simulink model "STANLEY"  (R2022b)
settings: Solver=ode15s  StartTime=0.0  StopTime=90  FixedStep=0.01  MaxStep=1e-2  MinStep=1e-3  RelTol=5e-3
PreLoadFcn:
  | %centerToFront = 1.4;
  | %centerToRear = 1.4;
values from neighbouring files (symbols this model uses):
  costmap = vehicleCostmap(costmapStruct.Costs,          'FreeThreshold',     costmapStruct.FreeThreshold,          'OccupiedThreshold', costmapStruct.OccupiedThreshold,          'MapLocation',       costmapStruct.MapExtent([1, 3]),          'CellSize',          costmapStruct.CellSize,          'CollisionChecker',  ccConfig)    [VisualizeBicyclePath.m]    (also in createParkingLotCostmap.m = vehicleCostmap(combinedMap,      'CellSize', cellSize,      )
  routePlan = table2struct(routePlan)    [RouteSupervisor.m]
undefined symbols (not defined in the file or in its folder): initialPose
libraries: drivingvehiclecontroller x2, simulink x2, simulink_extras x2, drivinglib x2, autolibshared x1
settings Model: Creator=emanuela  LastModifiedBy=emanuela
settings DataIOCC: SaveFinalState=on  SaveState=on  ReturnWorkspaceOutputs=off

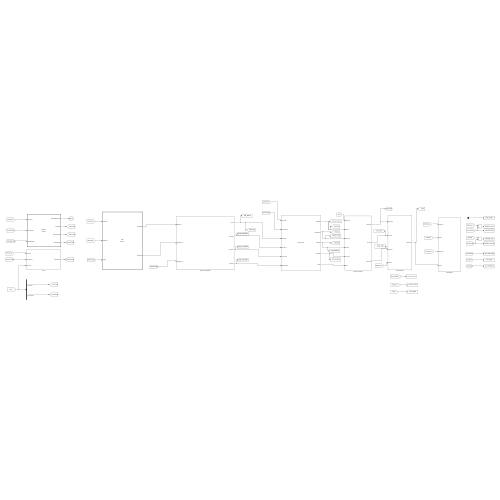
[thumbnail: Simulink's stored preview of the top-level diagram]
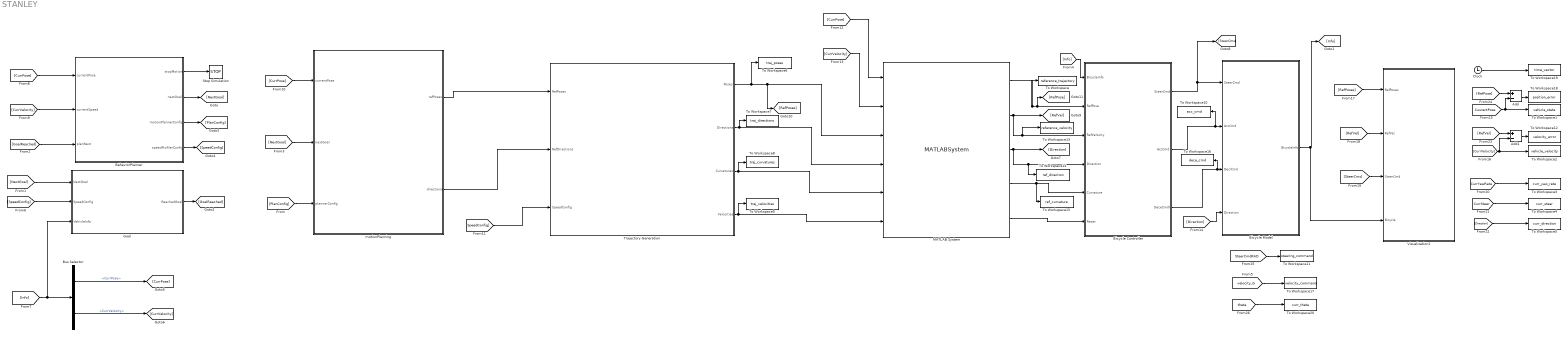
== system STANLEY ==
  Add : Sum  Inputs=+-
  Add1 : Sum  Inputs=+-
  BehaviorPlanner : MATLAB Function  TreatAsAtomicUnit=on  mask{Costmap=costmap, RoutePlan=routePlan, StartSpeed=0}
      mask prompts: Costmap "Vehicle costmap:"; RoutePlan "Route plan:"; StartSpeed "Initial vehicle speed  [m/s]:"
      mask init:
      | validateattributes(Costmap, {'vehicleCostmap'}, {'scalar'});
      | validateattributes(RoutePlan, {'table'}, {'ncols', 3});
      | validateattributes(StartSpeed, {'double'}, {'scalar','nonnegative'})
      | 
      | routePlanStruct   = table2struct(RoutePlan);
      | startPose         = routePlanStruct(1).StartPose;
      | 
      | varagout          = helperSLCreateUtilityStruct(Costmap);
      | vehicleDimsStruct = varagout{1};
      | costmapStruct     = varagout{2};
  Bicycle Controller : Subsystem
  Bicycle Model : Subsystem
  Bus Selector : BusSelector  OutputSignals=CurrPose,CurrVelocity
  Clock : Clock
  Goal : Subsystem
  MATLAB System : MATLABSystem  System=PathTracker  Wheelbase=2.8  HasResetOutput=on  SimulateUsing=Code generation
      mask Type: PathTracker
      mask Display:
      | disp('Path Tracker');
      | port_label('input',1,'CurrPose');
      | port_label('input',2,'CurrVelocity');
      | port_label('input',3,'RefPoses');
      | port_label('input',4,'Directions');
      | port_label('input',5,'Curvatures');
      | port_label('input',6,'RefVelocities');
      | port_label('output',1,'RefPose');
      | port_label('output',2,'RefVelocity');
      | port_label('output',3,'Direction');
      | port_label('output',4,'Curvature');
      | port_label('output',5,'Reset');
  Stop Simulation : Stop
  To Workspace : ToWorkspace  VariableName=reference_trajectory  SaveFormat=Timeseries  SampleTime=-1
  To Workspace1 : ToWorkspace  VariableName=vehicle_state  SaveFormat=Timeseries  SampleTime=-1
  To Workspace10 : ToWorkspace  VariableName=acc_cmd  SaveFormat=Timeseries  SampleTime=-1
  To Workspace11 : ToWorkspace  VariableName=steering_command  SaveFormat=Timeseries  SampleTime=-1
  To Workspace12 : ToWorkspace  VariableName=velocity_error  SaveFormat=Timeseries  SampleTime=-1
  To Workspace13 : ToWorkspace  VariableName=reference_velocity  SaveFormat=Timeseries  SampleTime=-1
  To Workspace14 : ToWorkspace  VariableName=ref_direction  SaveFormat=Timeseries  SampleTime=-1
  To Workspace15 : ToWorkspace  VariableName=ref_curvature  SaveFormat=Timeseries  SampleTime=-1
  To Workspace16 : ToWorkspace  VariableName=dece_cmd  SaveFormat=Timeseries  SampleTime=-1
  To Workspace17 : ToWorkspace  VariableName=velocity_command  SaveFormat=Timeseries  SampleTime=-1
  To Workspace18 : ToWorkspace  VariableName=position_error  SaveFormat=Timeseries  SampleTime=-1
  To Workspace19 : ToWorkspace  VariableName=time_vector  SampleTime=-1
  To Workspace2 : ToWorkspace  VariableName=vehicle_velocity  SaveFormat=Timeseries  SampleTime=-1
  To Workspace20 : ToWorkspace  VariableName=curr_theta  SaveFormat=Timeseries  SampleTime=-1
  To Workspace3 : ToWorkspace  VariableName=curr_yaw_rate  SaveFormat=Timeseries  SampleTime=-1
  To Workspace4 : ToWorkspace  VariableName=curr_steer  SaveFormat=Timeseries  SampleTime=-1
  To Workspace5 : ToWorkspace  VariableName=curr_direction  SaveFormat=Timeseries  SampleTime=-1
  To Workspace6 : ToWorkspace  VariableName=traj_poses  SaveFormat=Timeseries  SampleTime=-1
  To Workspace7 : ToWorkspace  VariableName=traj_directions  SaveFormat=Timeseries  SampleTime=-1
  To Workspace8 : ToWorkspace  VariableName=traj_curvatures  SaveFormat=Timeseries  SampleTime=-1
  To Workspace9 : ToWorkspace  VariableName=traj_velocities  SaveFormat=Timeseries  SampleTime=-1
  Trajectory Generation : Subsystem
  Visualization1 : Subsystem  mask{Costmap=costmap}
      mask prompts: Costmap "Vehicle costmap:"
      mask init:
      | validateattributes(Costmap, {'vehicleCostmap'}, {'scalar'});
      | 
      | varagout          = helperSLCreateUtilityStruct(Costmap);
      | vehicleDimsStruct = varagout{1};
      | costmapStruct     = varagout{2};
      mask DialogControl DescTextVar Prompt: Visualize simulation results.
  motionPlanning : MATLAB Function  TreatAsAtomicUnit=on  mask{Costmap=costmap}
      mask prompts: Costmap "Vehicle costmap:"
      mask init:
      | validateattributes(Costmap, {'vehicleCostmap'}, {'scalar'});
      | 
      | varagout          = helperSLCreateUtilityStruct(Costmap);
      | vehicleDimsStruct = varagout{1};
      | costmapStruct     = varagout{2};
  wires:
  Bicycle Model/1(BicycleInfo) -> Visualization1/4(Bicycle), [Info]
  [Info] -> Bicycle Controller/1(BicycleInfo)
  [NextGoal] -> Goal/1(NextGoal)
  BehaviorPlanner/2(nextGoal) -> [NextGoal]
  BehaviorPlanner/1(stopMotion) -> Stop Simulation/1
  [GoalReached] -> BehaviorPlanner/3(planNext)
  Goal/1(ReachedGoal) -> [GoalReached]
  [NextGoal] -> motionPlanning/2(nextGoal)
  BehaviorPlanner/3(motionPlannerConfig) -> [PlanConfig]
  [PlanConfig] -> motionPlanning/3(plannerConfig)
  BehaviorPlanner/4(speedProfilerConfig) -> [SpeedConfig]
  [SpeedConfig] -> Goal/2(SpeedConfig)
  Bus Selector/1 -> [CurrPose]  "<CurrPose>"
  Bus Selector/2 -> [CurrVelocity]  "<CurrVelocity>"
  [Info] -> Goal/3(VehicleInfo), Bus Selector/1
  [CurrPose] -> BehaviorPlanner/1(currentPose)
  [CurrVelocity] -> BehaviorPlanner/2(currentSpeed)
  [CurrPose] -> motionPlanning/1(currentPose)
  motionPlanning/1(refPoses) -> Trajectory Generation/1(RefPoses)
  motionPlanning/2(directions) -> Trajectory Generation/2(RefDirections)
  [SpeedConfig] -> Trajectory Generation/3(SpeedConfig)
  [CurrPose] -> MATLAB System/1
  [CurrVelocity] -> MATLAB System/2
  Trajectory Generation/2(Directions) -> To Workspace7/1, MATLAB System/4
  Trajectory Generation/3(Curvatures) -> To Workspace8/1, MATLAB System/5
  Trajectory Generation/4(Velocities) -> To Workspace9/1, MATLAB System/6
  MATLAB System/1 -> Bicycle Controller/2(RefPose), [RefPose], To Workspace/1
  MATLAB System/2 -> To Workspace13/1, Bicycle Controller/3(RefVelocity), [RefVel]
  MATLAB System/3 -> [Direction], To Workspace14/1, Bicycle Controller/4(Direction)
  MATLAB System/4 -> To Workspace15/1, Bicycle Controller/5(Curvature)
  Bicycle Controller/1(SteerCmd) -> [SteerCms], Bicycle Model/1(SteerCmd)
  Bicycle Controller/2(AccCmd) -> To Workspace10/1, Bicycle Model/2(AccCmd)
  Bicycle Controller/3(DeceCmdl) -> To Workspace16/1, Bicycle Model/3(DeclCmd)
  [Direction] -> Bicycle Model/4(Direction)
  Trajectory Generation/1(Poses) -> To Workspace6/1, [RefPoses], MATLAB System/3
  MATLAB System/5 -> Bicycle Controller/6(Reset)
  [RefPoses] -> Visualization1/1(RefPoses)
  [RefVel] -> Visualization1/2(RefVel)
  [SteerCms] -> Visualization1/3(SteerCmd)
  [CuurentPose] -> Add/2, To Workspace1/1
  [CurrVelocity] -> Add1/2, To Workspace2/1
  [CurrYawRate] -> To Workspace3/1
  [CurrSteer] -> To Workspace4/1
  [Direction] -> To Workspace5/1
  [RefVel] -> Add1/1
  [RefPose] -> Add/1
  Add1/1 -> To Workspace12/1
  Add/1 -> To Workspace18/1
  Clock/1 -> To Workspace19/1
  [SteerCmdRAD] -> To Workspace11/1
  [velocity_G] -> To Workspace17/1
  [theta] -> To Workspace20/1

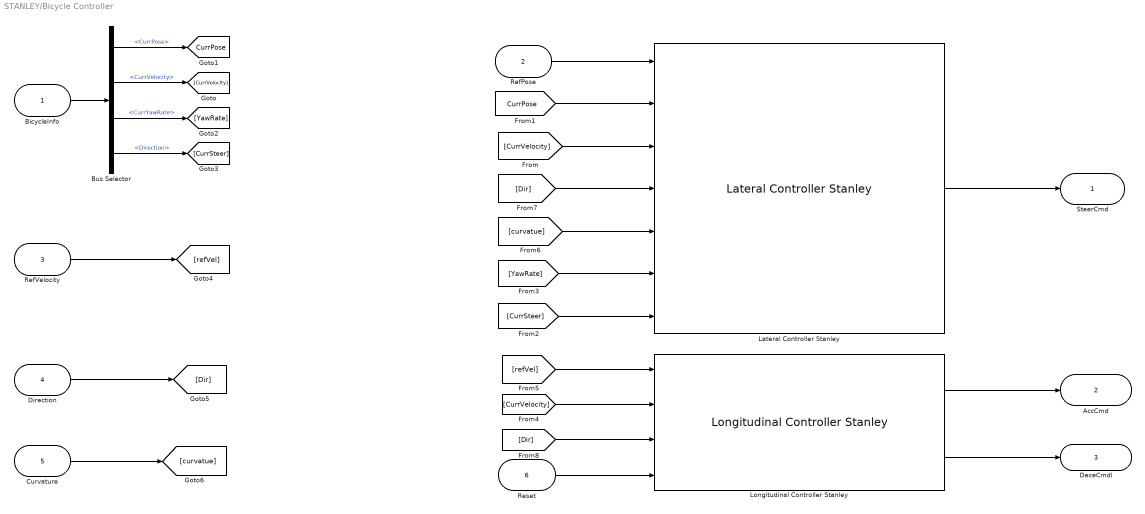
== system STANLEY/Bicycle Controller ==
  BicycleInfo : Inport
  RefPose : Inport  Port=2
  RefVelocity : Inport  Port=3
  Direction : Inport  Port=4
  Curvature : Inport  Port=5
  Reset : Inport  Port=6
  Bus Selector : BusSelector  OutputSignals=CurrPose,CurrVelocity,CurrYawRate,Direction
  Lateral Controller Stanley : drivingvehiclecontroller/Lateral Controller Stanley  ModelType=Dynamic bicycle model  PositionGainF=2  PositionGainR=2.5  YawRateGain=0.25  DelayGain=0.2  VehicleMass=1575  Lf=1.4  Lr=1.4  TireStiffness=19000  Wheelbase=2.8  MaxSteeringAngle=35
  Longitudinal Controller Stanley : drivingvehiclecontroller/Longitudinal Controller Stanley  Kp=2.5  Ki=1  SampleTime=0.01  MaxAcceleration=3  MaxDeceleration=6
  SteerCmd : Outport
  AccCmd : Outport  Port=2
  DeceCmdl : Outport  Port=3
  tag scope: CurrPose=global
  wires:
  BicycleInfo/1 -> Bus Selector/1
  Reset/1 -> Longitudinal Controller Stanley/4
  Lateral Controller Stanley/1 -> SteerCmd/1
  [CurrPose] -> Lateral Controller Stanley/2
  [YawRate] -> Lateral Controller Stanley/6
  [refVel] -> Longitudinal Controller Stanley/1
  [curvatue] -> Lateral Controller Stanley/5
  Longitudinal Controller Stanley/1 -> AccCmd/1
  Longitudinal Controller Stanley/2 -> DeceCmdl/1
  Bus Selector/1 -> [CurrPose]  "<CurrPose>"
  Bus Selector/2 -> [CurrVelocity]  "<CurrVelocity>"
  Bus Selector/3 -> [YawRate]  "<CurrYawRate>"
  Bus Selector/4 -> [CurrSteer]  "<Direction>"
  [CurrSteer] -> Lateral Controller Stanley/7
  [CurrVelocity] -> Lateral Controller Stanley/3
  [CurrVelocity] -> Longitudinal Controller Stanley/2
  RefVelocity/1 -> [refVel]
  Direction/1 -> [Dir]
  [Dir] -> Lateral Controller Stanley/4
  [Dir] -> Longitudinal Controller Stanley/3
  Curvature/1 -> [curvatue]
  RefPose/1 -> Lateral Controller Stanley/1

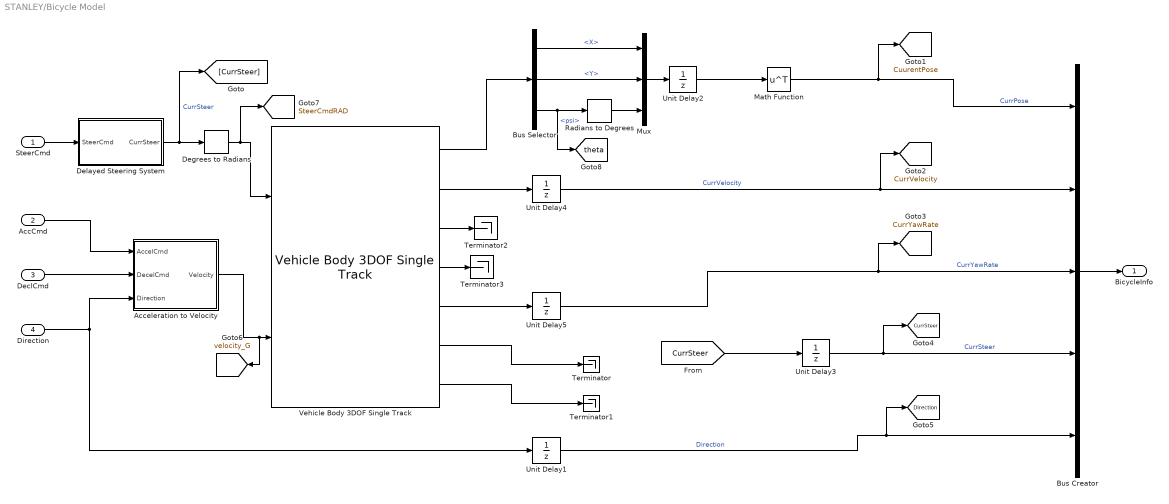
== system STANLEY/Bicycle Model ==
  SteerCmd : Inport
  AccCmd : Inport  Port=2
  DeclCmd : Inport  Port=3
  Direction : Inport  Port=4
  Acceleration to Velocity : Subsystem  TreatAsAtomicUnit=on
  Bus Creator : BusCreator  Inputs=5  OutDataTypeStr=Bus: vehicleInfoBus  NonVirtualBus=on
  Bus Selector : BusSelector  OutputSignals=InertFrm.RearAxl.Disp.X,InertFrm.RearAxl.Disp.Y,InertFrm.Cg.Ang.psi
  Degrees to Radians : simulink_extras/Transformations/Degrees to Radians
  Delayed Steering System : Subsystem
  Math Function : Math  Operator=transpose  SignedPower=on
  Mux : Mux  Inputs=3
  Radians to Degrees : simulink_extras/Transformations/Radians to Degrees
  Terminator{,1..3} (4 alike) : Terminator
  Unit Delay1 : UnitDelay  InitialCondition=1  SampleTime=-1  HasFrameUpgradeWarning=on
  Unit Delay2 : UnitDelay  InitialCondition=initialPose  SampleTime=-1  HasFrameUpgradeWarning=on
  Unit Delay3 : UnitDelay  SampleTime=-1  HasFrameUpgradeWarning=on
  Unit Delay4 : UnitDelay  SampleTime=-1  HasFrameUpgradeWarning=on
  Unit Delay5 : UnitDelay  SampleTime=-1  HasFrameUpgradeWarning=on
  Vehicle Body 3DOF Single Track : autolibshared/Vehicle Body 3DOF Single Track  trackMode=Single (bicycle)  inputMode=External longitudinal velocity  frontSteerMode=on  rearSteerMode=off  windMode=off  muMode=off  extFMode=off  extMMode=off  htchFMode=off  htchMMode=off  extXo=off  extpsio=off  extxdoto=off  extro=off  extYo=off  extTamb=off  extydoto=off  aMode=2  NF=2  NR=2  m=2000  a=1.4  b=1.6  h=0.35  dh=1  hh=0.2  X_o=13.1500  xdot_o=0  CalphaMode=off  sigmaMode=on  d=0  hl=0  w=[1.4,1.4]  Cy_f=12e3  Cy_r=11e3  sigma_f=.1  sigma_r=.1  alpha_f_brk=[-.1 .1]  Cy_f_data=[-9e3 9e3]  alpha_r_brk=[-.1 .1]  Cy_r_data=[-9e3 9e3]  Y_o=93.6500  ydot_o=0  Izz=4000  psi_o=0  r_o=0  Af=2  Cd=.3  Cl=.1  Cpm=.1  beta_w=[0 0.01:0.01:0.3]  Cs=[0 0.01:0.01:0.3]  Cym=[0 1e-6:0.01:0.3]  Pabs=101325  Tair=273  g=9.81  mu=1  xdot_tol=.01  Fznom=5000  Fxtire_sat=7e4  Fytire_sat=7e4  longOff=0  latOff=0  vertOff=0  wrapAng=off
  BicycleInfo : Outport  VectorParamsAs1DForOutWhenUnconnected=off
  tag scope: CurrSteer=global, CurrVelocity=global, CurrYawRate=global, CuurentPose=global, Direction=global, SteerCmdRAD=global, theta=global, velocity_G=global
  wires:
  Vehicle Body 3DOF Single Track/6 -> Terminator/1
  Vehicle Body 3DOF Single Track/7 -> Terminator1/1
  SteerCmd/1 -> Delayed Steering System/1(SteerCmd)
  Delayed Steering System/1(CurrSteer) -> [CurrSteer], Degrees to Radians/1  "CurrSteer"
  Degrees to Radians/1 -> [SteerCmdRAD], Vehicle Body 3DOF Single Track/1
  AccCmd/1 -> Acceleration to Velocity/1(AccelCmd)
  DeclCmd/1 -> Acceleration to Velocity/2(DecelCmd)
  Acceleration to Velocity/1(Velocity) -> [velocity_G], Vehicle Body 3DOF Single Track/2
  Vehicle Body 3DOF Single Track/1 -> Bus Selector/1
  Bus Selector/2 -> Mux/2  "<Y>"
  Unit Delay2/1 -> Math Function/1
  Bus Selector/1 -> Mux/1  "<X>"
  Mux/1 -> Unit Delay2/1
  Math Function/1 -> [CuurentPose], Bus Creator/1  "CurrPose"
  Bus Selector/3 -> [theta], Radians to Degrees/1  "<psi>"
  Radians to Degrees/1 -> Mux/3
  Vehicle Body 3DOF Single Track/3 -> Terminator2/1
  Vehicle Body 3DOF Single Track/2 -> Unit Delay4/1
  Vehicle Body 3DOF Single Track/4 -> Terminator3/1
  Vehicle Body 3DOF Single Track/5 -> Unit Delay5/1
  Direction/1 -> Unit Delay1/1, Acceleration to Velocity/3(Direction)
  Bus Creator/1 -> BicycleInfo/1
  [CurrSteer] -> Unit Delay3/1
  Unit Delay4/1 -> [CurrVelocity], Bus Creator/2  "CurrVelocity"
  Unit Delay5/1 -> [CurrYawRate], Bus Creator/3  "CurrYawRate"
  Unit Delay1/1 -> [Direction], Bus Creator/5  "Direction"
  Unit Delay3/1 -> [CurrSteer], Bus Creator/4  "CurrSteer"

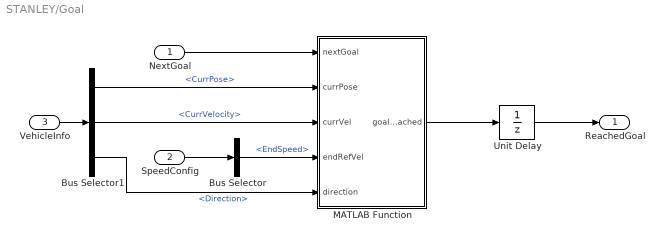
== system STANLEY/Goal ==
  NextGoal : Inport
  SpeedConfig : Inport  Port=2
  VehicleInfo : Inport  Port=3
  Bus Selector : BusSelector  OutputSignals=EndSpeed
  Bus Selector1 : BusSelector  OutputSignals=CurrPose,CurrVelocity,Direction
  MATLAB Function : MATLAB Function  TreatAsAtomicUnit=on
  Unit Delay : UnitDelay  SampleTime=-1  HasFrameUpgradeWarning=on
  ReachedGoal : Outport  VectorParamsAs1DForOutWhenUnconnected=off
  wires:
  Bus Selector/1 -> MATLAB Function/4(endRefVel)  "<EndSpeed>"
  Bus Selector1/1 -> MATLAB Function/2(currPose)  "<CurrPose>"
  VehicleInfo/1 -> Bus Selector1/1
  Unit Delay/1 -> ReachedGoal/1
  Bus Selector1/2 -> MATLAB Function/3(currVel)  "<CurrVelocity>"
  MATLAB Function/1(goalReached) -> Unit Delay/1
  SpeedConfig/1 -> Bus Selector/1
  Bus Selector1/3 -> MATLAB Function/5(direction)  "<Direction>"
  NextGoal/1 -> MATLAB Function/1(nextGoal)

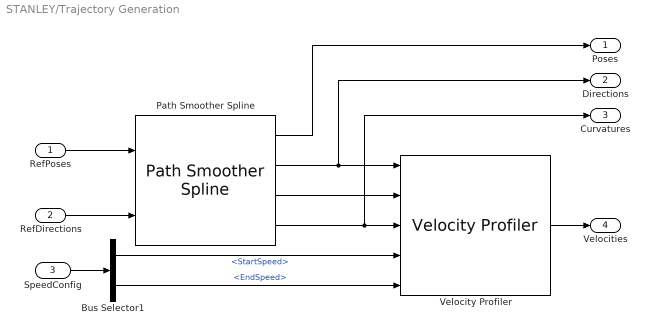
== system STANLEY/Trajectory Generation ==
  RefPoses : Inport
  RefDirections : Inport  Port=2
  SpeedConfig : Inport  Port=3
  Bus Selector1 : BusSelector  OutputSignals=StartSpeed,EndSpeed
  Path Smoother Spline : drivinglib/Path Smoother Spline  NumSmoothPoses=500  MinSeparation=1e-3  SampleTime=-1  ShowOptionalOutports=on  SimulateUsing=Interpreted execution
  Velocity Profiler : drivinglib/Velocity Profiler  MaxLongitudinalAccel=2  MaxLongitudinalDecel=4  MaxSpeed=10  MaxLongitudinalJerk=1  MaxLateralAccel=2  ShowOptionalOutport=off  SampleTime=-1  SimulateUsing=Interpreted execution
  Poses : Outport  VectorParamsAs1DForOutWhenUnconnected=off
  Directions : Outport  Port=2  VectorParamsAs1DForOutWhenUnconnected=off
  Curvatures : Outport  Port=3  VectorParamsAs1DForOutWhenUnconnected=off
  Velocities : Outport  Port=4  VectorParamsAs1DForOutWhenUnconnected=off
  wires:
  Velocity Profiler/1 -> Velocities/1
  Path Smoother Spline/2 -> Directions/1, Velocity Profiler/1
  Path Smoother Spline/4 -> Curvatures/1, Velocity Profiler/3
  Bus Selector1/2 -> Velocity Profiler/5  "<EndSpeed>"
  RefPoses/1 -> Path Smoother Spline/1
  SpeedConfig/1 -> Bus Selector1/1
  Bus Selector1/1 -> Velocity Profiler/4  "<StartSpeed>"
  Path Smoother Spline/3 -> Velocity Profiler/2
  RefDirections/1 -> Path Smoother Spline/2
  Path Smoother Spline/1 -> Poses/1

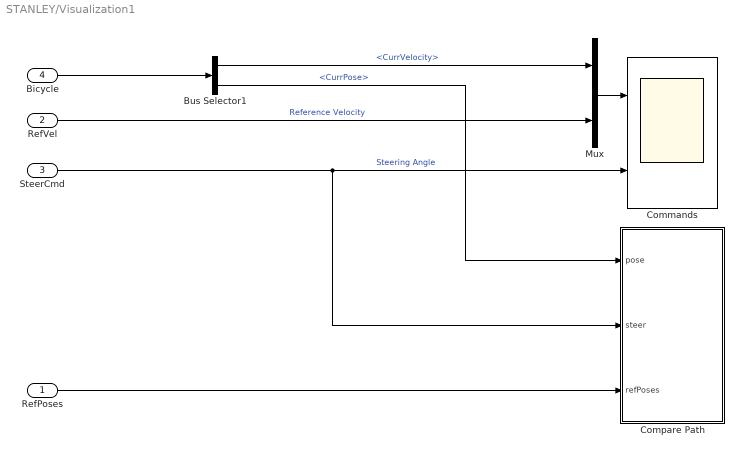
== system STANLEY/Visualization1 ==
  RefPoses : Inport
  RefVel : Inport  Port=2
  SteerCmd : Inport  Port=3
  Bicycle : Inport  Port=4
  Bus Selector1 : BusSelector  OutputSignals=CurrVelocity,CurrPose
  Commands : Scope  NumInputPorts=2
  Compare Path : MATLAB Function  TreatAsAtomicUnit=on
  Mux : Mux  Inputs=2
  wires:
  RefPoses/1 -> Compare Path/3(refPoses)
  Bus Selector1/1 -> Mux/1  "<CurrVelocity>"
  Bus Selector1/2 -> Compare Path/1(pose)  "<CurrPose>"
  RefVel/1 -> Mux/2  "Reference Velocity"
  Mux/1 -> Commands/1
  SteerCmd/1 -> Compare Path/2(steer), Commands/2  "Steering Angle"
  Bicycle/1 -> Bus Selector1/1

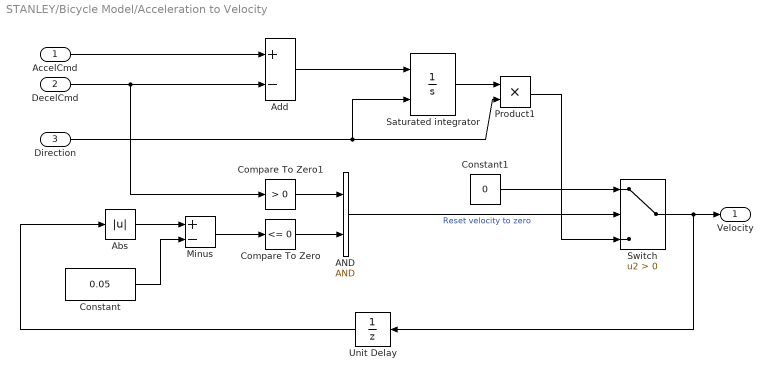
== system STANLEY/Bicycle Model/Acceleration to Velocity ==
  AccelCmd : Inport  PortDimensions=[1 1]
  DecelCmd : Inport  Port=2  PortDimensions=[1 1]
  Direction : Inport  Port=3
  AND : Logic  IconShape=distinctive  AllPortsSameDT=off  OutDataTypeStr=boolean
  Abs : Abs  SaturateOnIntegerOverflow=off
  Add : Sum  Inputs=+-
  Compare To Zero : simulink/Logic and Bit Operations/Compare To Zero  relop=<=  OutDataTypeStr=boolean
  Compare To Zero1 : simulink/Logic and Bit Operations/Compare To Zero  relop=>  OutDataTypeStr=boolean
  Constant : Constant  Value=0.05
  Constant1 : Constant  Value=0
  Minus : Sum  Inputs=+-
  Product1 : Product
  Saturated integrator : Integrator  ExternalReset=either  LimitOutput=on  LowerSaturationLimit=0  AbsoluteTolerance=1e-3  ZeroCross=off
  Switch : Switch  Criteria=u2 > Threshold  SaturateOnIntegerOverflow=off  InputSameDT=off
  Unit Delay : UnitDelay  SampleTime=-1  HasFrameUpgradeWarning=on
  Velocity : Outport  VectorParamsAs1DForOutWhenUnconnected=off
  wires:
  Direction/1 -> Product1/2, Saturated integrator/2
  AccelCmd/1 -> Add/1
  Add/1 -> Saturated integrator/1
  DecelCmd/1 -> Compare To Zero1/1, Add/2
  Unit Delay/1 -> Abs/1
  Abs/1 -> Minus/1
  Constant/1 -> Minus/2
  Minus/1 -> Compare To Zero/1
  Compare To Zero/1 -> AND/2
  Compare To Zero1/1 -> AND/1
  AND/1 -> Switch/2  "Reset velocity to zero"
  Switch/1 -> Unit Delay/1, Velocity/1
  Constant1/1 -> Switch/1
  Saturated integrator/1 -> Product1/1
  Product1/1 -> Switch/3

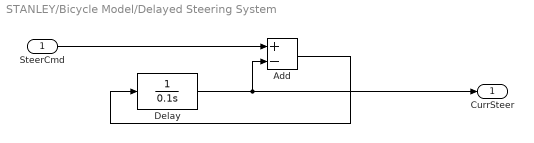
== system STANLEY/Bicycle Model/Delayed Steering System ==
  SteerCmd : Inport
  Add : Sum  Inputs=+-
  Delay : TransferFcn  Denominator=[0.1 0]
  CurrSteer : Outport  VectorParamsAs1DForOutWhenUnconnected=off
  wires:
  Add/1 -> Delay/1
  SteerCmd/1 -> Add/1
  Delay/1 -> CurrSteer/1, Add/2

== matlab function STANLEY/Visualization1/Compare Path ==
  settings: updateMethod=DISCRETE  sampleTime=0.1
  data: pose input size=[1 3]; steer input; refPoses input; costmapStruct parameter; vehicleDimsStruct parameter
function visualizePath(pose, steer, refPoses, costmapStruct, vehicleDimsStruct)

%visualizePath Display simulation results.

coder.extrinsic('VisualizeBicyclePath');

VisualizeBicyclePath(pose, steer, refPoses, costmapStruct, vehicleDimsStruct);
end

== matlab function STANLEY/motionPlanning ==
  settings: updateMethod=DISCRETE  sampleTime=0.1
  data: refPoses output size=[100 3]; currentPose input size=[1 3]; nextGoal input size=[1 3]; plannerConfig input Bus: plannerConfigBus; costmapStruct parameter; vehicleDimsStruct parameter; directions output size=[100 1]
function [refPoses, directions] = motionPlanning(currentPose, nextGoal, ...
    plannerConfig, costmapStruct, vehicleDimsStruct)

%motionPlanning plan a feasible path using pathPlannerRRT.

%#codegen

persistent nextGoalPose posesInternal directionsInternal

% Initialize persistent variables
if isempty(nextGoalPose)
    nextGoalPose = [0 0 0];
end

if isempty(posesInternal)
    posesInternal = [0 0 0];
end

if isempty(directionsInternal)
    directionsInternal = 1;
end

% Create vehicleDimensions object
vehicleDims = vehicleDimensions( ...
    vehicleDimsStruct.Length, ...
    vehicleDimsStruct.Width, ...
    vehicleDimsStruct.Height, ...
    'Wheelbase',          vehicleDimsStruct.Wheelbase, ...
    'RearOverhang',       vehicleDimsStruct.RearOverhang, ...
    'WorldUnits',         char(vehicleDimsStruct.WorldUnits));

ccConfig = inflationCollisionChecker(vehicleDims, 4);

% Initialize vehicleCostmap object
costmap = vehicleCostmap(costmapStruct.Costs, ...
    'FreeThreshold',      costmapStruct.FreeThreshold, ...
    'OccupiedThreshold',  costmapStruct.OccupiedThreshold, ...
    'MapLocation',        costmapStruct.MapExtent([1, 3]), ...
    'CellSize',           costmapStruct.CellSize, ...
    'CollisionChecker',   ccConfig);

% Create pathPlannerRRT object
% motionPlanner = pathPlannerRRT(costmap, ...
%     'ConnectionDistance', plannerConfig.ConnectionDistance, ...
%     'MinIterations',      plannerConfig.MinIterations, ...
%     'GoalTolerance',      plannerConfig.GoalTolerance, ...
%     'MinTurningRadius',   plannerConfig.MinTurningRadius);

% Create pathPlannerRRT object
motionPlanner = pathPlannerRRT(costmap, ...
    'ConnectionDistance', 30.0, ... % Valore generoso dal tuo main.m
    'MinIterations',      2000, ... % Valore generoso dal tuo main.m
    'GoalTolerance',      [0.5 0.5 10], ...
    'MinTurningRadius',   4.0);

% Only plan the path if there is a new goal
if ~isequal(nextGoalPose, nextGoal)
    nextGoalPose  = nextGoal;
    vehiclePose   = currentPose;
    refPath       = plan(motionPlanner, vehiclePose, nextGoalPose);
    [refPoses, directions] = interpolate(refPath);
    posesInternal          = refPoses;
    directionsInternal     = directions;
else
    refPoses   = posesInternal;
    directions = directionsInternal;
end

if isempty(refPoses)
    error('No feasible path can be found.')
end

end

== matlab function STANLEY/Goal/MATLAB Function ==
  data: nextGoal input size=[1 3]; goalReached output size=[1 1]; currPose input size=[1 3]; currVel input size=[1 1]; endRefVel input size=[1 1]; direction input
function goalReached = GoalChecker(nextGoal, currPose, currVel, endRefVel, direction)
    
    goalReached = helperGoalChecker(nextGoal, currPose, currVel, endRefVel, direction);
end

== matlab function STANLEY/BehaviorPlanner ==
  settings: updateMethod=DISCRETE  sampleTime=0.1
  data: stopMotion output; nextGoal output double size=[1 3]; motionPlannerConfig output Bus: plannerConfigBus; speedProfilerConfig output Bus: speedConfigBus; routePlanStruct parameter; currentPose input size=[1 3]; currentSpeed input size=[1 1]; planNext input size=[1 1]; startPose parameter size=[1 3]; StartSpeed parameter
function [stopMotion, nextGoal, motionPlannerConfig, speedProfilerConfig] = manageParkingManeuvers(routePlanStruct, currentPose, currentSpeed, planNext, startPose, StartSpeed)
% manageParkingManeuvers: gestisce la sequenza di obiettivi di alto livello.
% Utilizza la classe personalizzata 'RouteSupervisor'.

% Pre-inizializza gli output per il Coder di Simulink
nextGoal     = coder.nullcopy(zeros(1, 3));
stopMotion   = coder.nullcopy(logical(0));

% Le variabili persistenti mantengono lo stato tra le chiamate
persistent routeManager
persistent nextGoalPose plannerConfig speedConfig

% Inizializzazione al primo passo della simulazione
if isempty(routeManager)
    
    % Inizializza l'oggetto che gestisce la rotta, usando la nostra classe personalizzata.
    steerLimit = 30; % Gradi
    routeManager = RouteSupervisor(routePlanStruct, steerLimit); 
    
    % Richiedi la prima manovra
    [nextGoalPose, plannerConfig, speedConfig] = requestManeuver(routeManager, startPose, StartSpeed);
end

% Se il Goal Checker segnala che il segmento è completo, richiedi la manovra successiva.
if planNext && ~reachedDestination(routeManager)
    [nextGoalPose, plannerConfig, speedConfig] = requestManeuver(routeManager, currentPose, currentSpeed);
end

% Logica per fermare il veicolo una volta arrivato a destinazione finale.
disTol = 1.0;
stopMotion = planNext && reachedDestination(routeManager) && ...
    norm(currentPose(1:2) - nextGoalPose(1:2)) < disTol;
    
% Assegna i valori alle porte di uscita del blocco
nextGoal            = nextGoalPose;
motionPlannerConfig = plannerConfig;
speedProfilerConfig = speedConfig;

end
